simulink model "final_output"  (R2024a)
settings: Solver=VariableStepAuto  StartTime=0.0  StopTime=2  MaxStep=1e-3  RelTol=1e-3  EnableMultiTasking=on
PreLoadFcn:
  | DualActiveBridgeConverterData
values from neighbouring files (symbols this model uses):
  C_HV = 0.0001    [matlab.mat]
  C_LV = 0.002    [matlab.mat]
  Cs_FET = inf    [matlab.mat]
  Fsw = 100000    [matlab.mat]
  Ki_Ireg = 500    [matlab.mat]
  Kp_Ireg = 0.1    [matlab.mat]
  L_Inductor = 1.5e-05    [matlab.mat]
  Lm_Tr = 0.00072    [matlab.mat]
  Lprim_Tr = 1.7e-05    [matlab.mat]
  Lsec_Tr = 0    [matlab.mat]
  N_Tr = 1.6    [matlab.mat]
  Pnom = 10000    [matlab.mat]
  R_DCsrc1 = 0.01    [matlab.mat]
  R_DCsrc2 = 0.05    [matlab.mat]
  R_Inductor = 0.016    [matlab.mat]
  RC_HV = 0.001    [matlab.mat]
  RC_LV = 0.001    [matlab.mat]
  Rm_Tr = 10000    [matlab.mat]
  Ron_Diode = 0.01    [matlab.mat]
  Ron_FET = 0.016    [matlab.mat]
  Rprim_Tr = 0.043    [matlab.mat]
  Rs_FET = 1000000    [matlab.mat]
  Rsec_Tr = 1e-06    [matlab.mat]
  Ts_Control = 1e-06    [matlab.mat]
  Vf_Diode = 4.2    [matlab.mat]
  Vnom_HV = 800    [matlab.mat]
  Vnom_LV = 450    [matlab.mat]
undefined symbols (not defined in the file or in its folder): DiscIntNeverNeededParam, Ion, Lithium
libraries: spsSeriesRLCBranchLib x14, spsDiodeLib x12, spsVoltageMeasurementLib x11, spsMosfetLib x9, spsCurrentMeasurementLib x8, spsIdealSwitchLib x8, powerlib_extras x5, spsMeanLib x5, spsRMSLib x3, simulink x3, spsThreePhaseVIMeasurementLib x2, spsUniversalBridgeLib x2
(part 2 of 2)

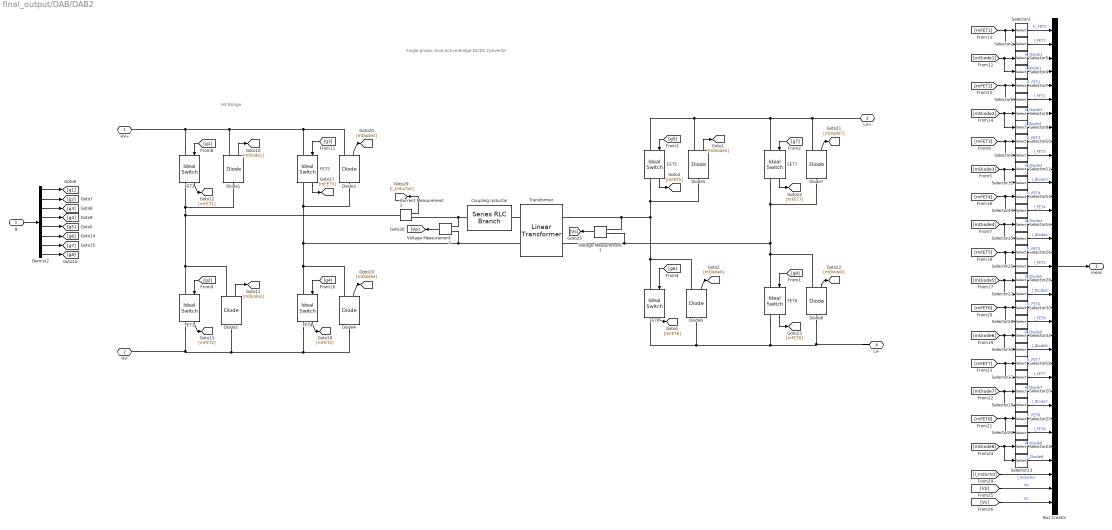
== system final_output/DAB/DAB2 ==
  note: HV Bridge
  note: Single-phase, Dual-Active Bridge
      | DC/DC Converter
  g : Inport  PortDimensions=8
  Bus Creator : BusCreator  Inputs=35
  Coupling Inductor : spsSeriesRLCBranchLib/Series RLC Branch  LConnTagsString=__new0  RConnTagsString=__new0  BranchType=RL  Resistance=R_Inductor  Inductance=L_Inductor  SetiL0=off  InitialCurrent=0  Capacitance=1e-6  Setx0=off  InitialVoltage=0  Measurements=None
  Current Measurement2 : spsCurrentMeasurementLib/Current Measurement  PhasorSimulation=off  OutputType=Complex  PSBequivalent=0
  Demux2 : Demux  Outputs=8
  Diode{1..8} (8 alike) : spsDiodeLib/Diode  Ron=Ron_Diode  Lon=0  Vf=Vf_Diode  IC=0  UseSnubber=0  Rs=inf  Cs=inf  Measurements=on
  FET{1..8} (8 alike) : spsIdealSwitchLib/Ideal Switch  Ron=Ron_FET  Lon=0  IC=0  Rs=Rs_FET  Cs=Cs_FET  Measurements=on
  Selector{1..2,4,6,8,11,13,15,17,19,21,23,25,27,29,31} (16 alike) : Selector  InputPortWidth=2  IndexOptions=Index vector (dialog)  Indices=1  OutputSizes=1
  Selector{3,5,7,9..10,12,14,16,18,20,22,24,26,28,30,32} (16 alike) : Selector  InputPortWidth=2  IndexOptions=Index vector (dialog)  Indices=2  OutputSizes=1
  Transformer : spsLinearTransformerLib/Linear Transformer  UNITS=SI  NominalPower="[ Param1_Tr(1),  Param1_Tr(2)]"  winding1="[ Param2_Tr(1),  Param2_Tr(2), Param2_Tr(3)]"  winding2="[ Param3_Tr(1),  Param3_Tr(2), Param3_Tr(3)]"  ThreeWindings=off  winding3=[3.15e+05 0.7938 0.084225]  RmLm="[ Param4_Tr(1),  Param4_Tr(2)]"  Measurements=None  DataType=on
  Voltage Measurement1 : spsVoltageMeasurementLib/Voltage Measurement  PhasorSimulation=off  OutputType=Complex  PSBequivalent=0
  Voltage Measurement2 : spsVoltageMeasurementLib/Voltage Measurement  PhasorSimulation=off  OutputType=Complex  PSBequivalent=0
  HV+ : PMIOPort  Side=Left
  HV- : PMIOPort  Port=2  Side=Left
  LV+ : PMIOPort  Port=3  Side=Right
  LV- : PMIOPort  Port=4  Side=Right
  meas : Outport  PortDimensions=35
  wires:
  Voltage Measurement2/1 -> [Vp]
  Demux2/8 -> [g8]
  Selector20/1 -> Bus Creator/27  "V_Diode7"
  Selector21/1 -> Bus Creator/30  "I_FET8"
  Selector22/1 -> Bus Creator/29  "V_FET8"
  Selector24/1 -> Bus Creator/31  "V_Diode8"
  [mDiode5] -> Selector27/1, Selector28/1
  Selector27/1 -> Bus Creator/20  "I_Diode5"
  [mFET6] -> Selector30/1, Selector29/1
  Selector23/1 -> Bus Creator/32  "I_Diode8"
  Selector32/1 -> Bus Creator/23  "V_Diode6"
  Selector26/1 -> Bus Creator/17  "V_FET5"
  Selector28/1 -> Bus Creator/19  "V_Diode5"
  Selector25/1 -> Bus Creator/18  "I_FET5"
  [mFET5] -> Selector25/1, Selector26/1
  FET3/1 -> [mFET3]
  Diode4/1 -> [mDiode4]
  FET4/1 -> [mFET4]
  Selector19/1 -> Bus Creator/28  "I_Diode7"
  FET7/1 -> [mFET7]
  Selector5/1 -> Bus Creator/3  "V_Diode1"
  [mDiode2] -> Selector8/1, Selector9/1
  [g4] -> FET4/1
  Selector4/1 -> Bus Creator/4  "I_Diode1"
  [mFET4] -> Selector14/1, Selector13/1
  Diode2/1 -> [mDiode2]
  Demux2/1 -> [g1]
  FET1/1 -> [mFET1]
  Selector18/1 -> Bus Creator/25  "V_FET7"
  Selector3/1 -> Bus Creator/1  "V_FET1"
  [mFET8] -> Selector21/1, Selector22/1
  FET2/1 -> [mFET2]
  [mDiode4] -> Selector16/1, Selector15/1
  [g1] -> FET1/1
  [g3] -> FET3/1
  Demux2/4 -> [g4]
  [mFET1] -> Selector3/1, Selector2/1
  Diode1/1 -> [mDiode1]
  Demux2/2 -> [g2]
  Diode6/1 -> [mDiode6]
  Demux2/3 -> [g3]
  Diode5/1 -> [mDiode5]
  [mDiode1] -> Selector5/1, Selector4/1
  Diode3/1 -> [mDiode3]
  Demux2/7 -> [g7]
  Selector6/1 -> Bus Creator/6  "I_FET2"
  Selector2/1 -> Bus Creator/2  "I_FET1"
  [mDiode3] -> Selector11/1, Selector12/1
  Selector13/1 -> Bus Creator/14  "I_FET4"
  Selector10/1 -> Bus Creator/9  "V_FET3"
  [mFET3] -> Selector1/1, Selector10/1
  Selector15/1 -> Bus Creator/16  "I_Diode4"
  Selector16/1 -> Bus Creator/15  "V_Diode4"
  Selector14/1 -> Bus Creator/13  "V_FET4"
  Selector30/1 -> Bus Creator/21  "V_FET6"
  [g7] -> FET7/1
  Demux2/6 -> [g6]
  [g8] -> FET8/1
  Selector9/1 -> Bus Creator/7  "V_Diode2"
  [g2] -> FET2/1
  FET6/1 -> [mFET6]
  Diode7/1 -> [mDiode7]
  [mDiode7] -> Selector20/1, Selector19/1
  Selector11/1 -> Bus Creator/12  "I_Diode3"
  Selector29/1 -> Bus Creator/22  "I_FET6"
  [mFET2] -> Selector6/1, Selector7/1
  [mDiode8] -> Selector23/1, Selector24/1
  Diode8/1 -> [mDiode8]
  FET5/1 -> [mFET5]
  Selector17/1 -> Bus Creator/26  "I_FET7"
  Selector12/1 -> Bus Creator/11  "V_Diode3"
  Current Measurement2/1 -> [I_Inductor]
  Selector1/1 -> Bus Creator/10  "I_FET3"
  Demux2/5 -> [g5]
  Selector31/1 -> Bus Creator/24  "I_Diode6"
  [mFET7] -> Selector18/1, Selector17/1
  Selector8/1 -> Bus Creator/8  "I_Diode2"
  [g5] -> FET5/1
  Selector7/1 -> Bus Creator/5  "V_FET2"
  FET8/1 -> [mFET8]
  [mDiode6] -> Selector32/1, Selector31/1
  [g6] -> FET6/1
  g/1 -> Demux2/1
  Bus Creator/1 -> meas/1
  Voltage Measurement1/1 -> [Vs]
  [I_Inductor] -> Bus Creator/33  "I_Inductor"
  [Vp] -> Bus Creator/34  "Vp"
  [Vs] -> Bus Creator/35  "Vs"
  connections:
  FET7/LConn1 -- LV+/RConn1 -- Diode7/RConn1 -- Diode5/RConn1 -- FET5/LConn1
  FET1/LConn1 -- HV+/RConn1 -- Diode3/RConn1 -- FET3/LConn1 -- Diode1/RConn1
  FET2/RConn1 -- HV-/RConn1 -- FET4/RConn1 -- Diode4/LConn1 -- Diode2/LConn1
  Diode2/RConn1 -- Current Measurement2/LConn1 -- Diode1/LConn1 -- FET1/RConn1 -- FET2/LConn1
  Diode4/RConn1 -- FET4/LConn1 -- Transformer/LConn2 -- Voltage Measurement2/LConn2 -- FET3/RConn1 -- Diode3/LConn1
  FET6/RConn1 -- Diode6/LConn1 -- LV-/RConn1 -- Diode8/LConn1 -- FET8/RConn1
  FET7/RConn1 -- Voltage Measurement1/LConn2 -- Transformer/RConn2 -- FET8/LConn1 -- Diode8/RConn1 -- Diode7/LConn1
  FET6/LConn1 -- Voltage Measurement1/LConn1 -- Transformer/RConn1 -- Diode5/LConn1 -- FET5/RConn1 -- Diode6/RConn1
  Current Measurement2/RConn1 -- Voltage Measurement2/LConn1 -- Coupling Inductor/LConn1
  Transformer/LConn1 -- Coupling Inductor/RConn1

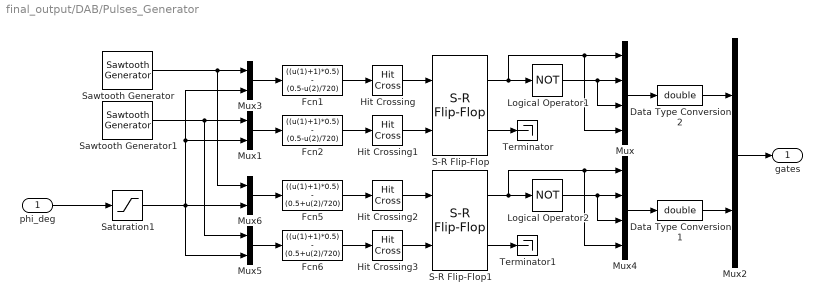
== system final_output/DAB/Pulses_Generator ==
  phi_deg : Inport
  Data Type Conversion1 : DataTypeConversion  OutDataTypeStr=double  SaturateOnIntegerOverflow=off  RndMeth=Floor
  Data Type Conversion2 : DataTypeConversion  OutDataTypeStr=double  SaturateOnIntegerOverflow=off  RndMeth=Floor
  Fcn1 : Fcn  Expr=((u(1)+1)*0.5) - (0.5-u(2)/720)
  Fcn2 : Fcn  Expr=((u(1)+1)*0.5) - (0.5-u(2)/720)
  Fcn5 : Fcn  Expr=((u(1)+1)*0.5) - (0.5+u(2)/720)
  Fcn6 : Fcn  Expr=((u(1)+1)*0.5) - (0.5+u(2)/720)
  Hit Crossing{,1..3} (4 alike) : HitCross  HitCrossingDirection=rising
  Logical Operator1 : Logic  Operator=NOT  AllPortsSameDT=off  OutDataTypeStr=boolean
  Logical Operator2 : Logic  Operator=NOT  AllPortsSameDT=off  OutDataTypeStr=boolean
  Mux : Mux
  Mux{1,3,5..6} (4 alike) : Mux  Inputs=2
  Mux2 : Mux  Inputs=[4,4]
  Mux4 : Mux
  S-R Flip-Flop : simulink_extras/Flip Flops/S-R Flip-Flop  initial_condition=0
  S-R Flip-Flop1 : simulink_extras/Flip Flops/S-R Flip-Flop  initial_condition=0
  Saturation1 : Saturate  UpperLimit=180  LowerLimit=-180
  Sawtooth Generator : spsSawtoothGeneratorLib/Sawtooth Generator  Freq=Fsw  Phase=0  Ts=0
  Sawtooth Generator1 : spsSawtoothGeneratorLib/Sawtooth Generator  Freq=Fsw  Phase=180  Ts=0
  Terminator : Terminator
  Terminator1 : Terminator
  gates : Outport
  wires:
  Mux2/1 -> gates/1
  Logical Operator1/1 -> Mux/2, Mux/3
  phi_deg/1 -> Saturation1/1
  Sawtooth Generator/1 -> Mux6/1, Mux3/1
  Fcn1/1 -> Hit Crossing/1
  Fcn2/1 -> Hit Crossing1/1
  Hit Crossing/1 -> S-R Flip-Flop/1
  Hit Crossing1/1 -> S-R Flip-Flop/2
  S-R Flip-Flop/1 -> Mux/4, Mux/1, Logical Operator1/1
  S-R Flip-Flop/2 -> Terminator/1
  Mux/1 -> Data Type Conversion2/1
  Data Type Conversion2/1 -> Mux2/1
  Data Type Conversion1/1 -> Mux2/2
  Mux3/1 -> Fcn1/1
  Mux1/1 -> Fcn2/1
  Sawtooth Generator1/1 -> Mux5/1, Mux1/1
  Saturation1/1 -> Mux6/2, Mux5/2, Mux1/2, Mux3/2
  Mux5/1 -> Fcn6/1
  Mux6/1 -> Fcn5/1
  Mux4/1 -> Data Type Conversion1/1
  S-R Flip-Flop1/2 -> Terminator1/1
  S-R Flip-Flop1/1 -> Logical Operator2/1, Mux4/1, Mux4/4
  Hit Crossing3/1 -> S-R Flip-Flop1/2
  Hit Crossing2/1 -> S-R Flip-Flop1/1
  Fcn6/1 -> Hit Crossing3/1
  Fcn5/1 -> Hit Crossing2/1
  Logical Operator2/1 -> Mux4/3, Mux4/2

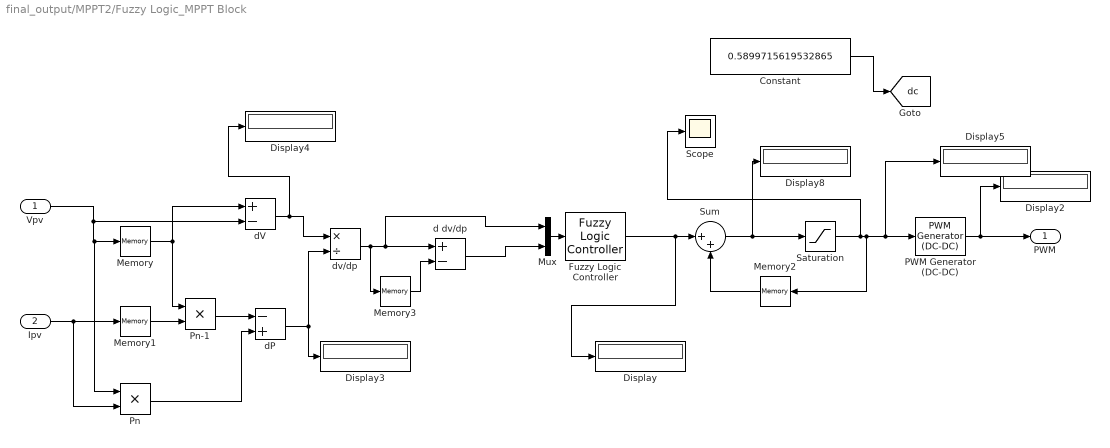
== system final_output/MPPT2/Fuzzy Logic_MPPT Block ==
  Vpv : Inport
  Ipv : Inport  Port=2
  Constant : Constant  Value=0.5899715619532865
  Display{,2..5,8} (6 alike) : Display
  Fuzzy Logic Controller : fuzblock/Fuzzy Logic  Controller  FIS='fuzzy_mppt.fis'  OutputSampleNumber=101  DataType=double  FuzzifiedInputs=off  RuleFiringStrengths=off  RuleOutputs=off  AggregatedOutputs=off  SimulateUsing=Interpreted execution  OutOfRangeInputValueMessage=warning  NoRuleFiredMessage=warning  EmptyOutputFuzzySetMessage=warning
  Memory{,1..3} (4 alike) : Memory  InheritSampleTime=on
  Mux : Mux  Inputs=2
  PWM Generator (DC-DC) : spsPWMGeneratorDCDCLib/PWM Generator (DC-DC)  Fsw=10000  Ts=0
  Pn : Product
  Pn-1 : Product
  Saturation : Saturate  UpperLimit=0.9  LowerLimit=0.1  OutDataTypeStr=double
  Scope : Scope
  Sum : Sum  Inputs=|++
  d dv/dp : Sum  Inputs=+-
  dP : Sum  Inputs=-+
  dV : Sum  Inputs=+-
  dv/dp : Product  Inputs=*/
  PWM : Outport  VectorParamsAs1DForOutWhenUnconnected=off
  tag scope: dc=global
  wires:
  Vpv/1 -> Memory/1, Pn/1, dV/2
  PWM Generator (DC-DC)/1 -> PWM/1, Display2/1
  Mux/1 -> Fuzzy Logic Controller/1
  Pn/1 -> dP/2
  Pn-1/1 -> dP/1
  Memory1/1 -> Pn-1/2
  Ipv/1 -> Memory1/1, Pn/2
  Memory/1 -> Pn-1/1, dV/1
  dV/1 -> Display4/1, dv/dp/1
  dP/1 -> dv/dp/2, Display3/1
  dv/dp/1 -> Memory3/1, Mux/1, d dv/dp/1
  Memory3/1 -> d dv/dp/2
  Memory2/1 -> Sum/2
  Sum/1 -> Display8/1, Saturation/1
  Constant/1 -> [dc]
  d dv/dp/1 -> Mux/2
  Saturation/1 -> Display5/1, PWM Generator (DC-DC)/1, Memory2/1, Scope/1
  Fuzzy Logic Controller/1 -> Sum/1, Display/1

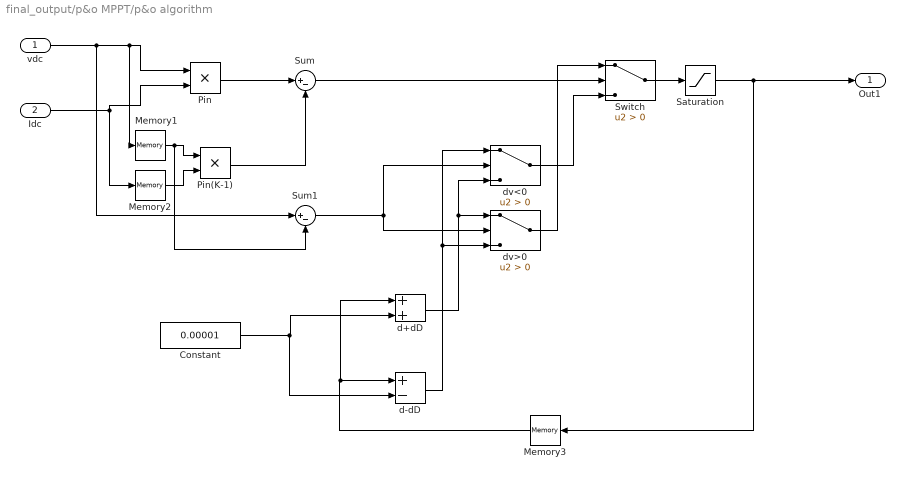
== system final_output/p&o MPPT/p&o algorithm ==
  vdc : Inport
  Idc : Inport  Port=2
  Constant : Constant  Value=0.00001
  Memory1 : Memory
  Memory2 : Memory
  Memory3 : Memory
  Pin : Product
  Pin(K-1) : Product
  Saturation : Saturate  UpperLimit=0.9  LowerLimit=0
  Sum : Sum  Inputs=|+-
  Sum1 : Sum  Inputs=|+-
  Switch : Switch  Criteria=u2 > Threshold  SaturateOnIntegerOverflow=off  InputSameDT=off
  d+dD : Sum
  d-dD : Sum  Inputs=+-
  dv<0 : Switch  Criteria=u2 > Threshold  SaturateOnIntegerOverflow=off  InputSameDT=off
  dv>0 : Switch  Criteria=u2 > Threshold  SaturateOnIntegerOverflow=off  InputSameDT=off
  Out1 : Outport
  wires:
  vdc/1 -> Sum1/1, Memory1/1, Pin/1
  Idc/1 -> Pin/2, Memory2/1
  Memory1/1 -> Sum1/2, Pin(K-1)/1
  Memory2/1 -> Pin(K-1)/2
  Pin/1 -> Sum/1
  Pin(K-1)/1 -> Sum/2
  Sum/1 -> Switch/2
  Sum1/1 -> dv<0/2, dv>0/2
  dv<0/1 -> Switch/3
  Memory3/1 -> d+dD/1, d-dD/1
  Switch/1 -> Saturation/1
  Constant/1 -> d-dD/2, d+dD/2
  d+dD/1 -> dv<0/3, dv>0/1
  d-dD/1 -> dv>0/3, dv<0/1
  dv>0/1 -> Switch/1
  Saturation/1 -> Memory3/1, Out1/1

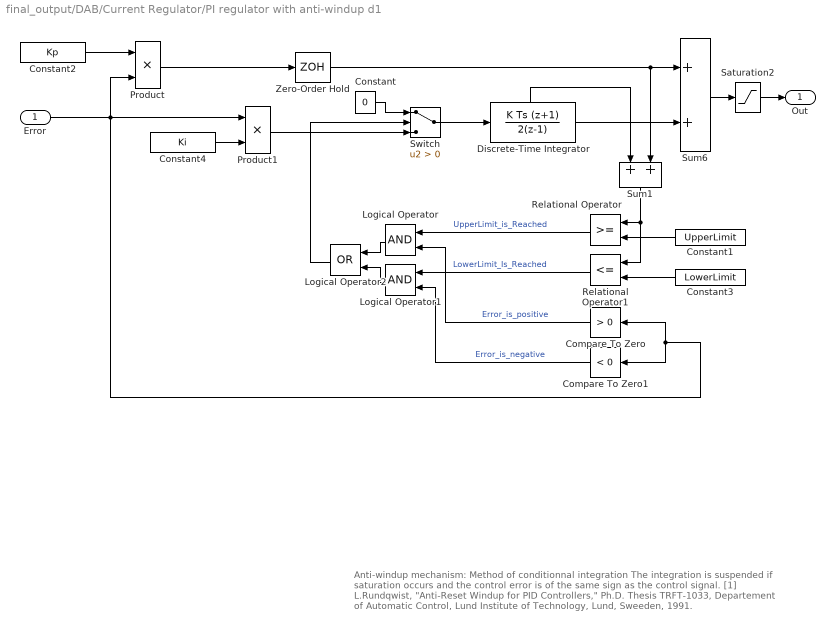
== system final_output/DAB/Current Regulator/PI regulator with anti-windup d1 ==
  note: Anti-windup mechanism: Method of conditionnal integration
      |
      | The integration is suspended if saturation occurs and the
      | control error is of the same sign as the control signal.
      |
      | [1] L.Rundqwist, "Anti-Reset Windup for PID Controllers," Ph.D. Thesis TRFT-1033,
      | Departement of Automatic Control, Lund Institute of Technology, Lund, Sweeden, 1991.
  Error : Inport  SampleTime=Ts
  Compare To Zero : simulink/Logic and Bit Operations/Compare To Zero  relop=>  OutDataTypeStr=uint8  ZeroCross=off
  Compare To Zero1 : simulink/Logic and Bit Operations/Compare To Zero  relop=<  OutDataTypeStr=uint8  ZeroCross=off
  Constant : Constant  Value=0
  Constant1 : Constant  Value=UpperLimit
  Constant2 : Constant  Value=Kp  SampleTime=Ts
  Constant3 : Constant  Value=LowerLimit
  Constant4 : Constant  Value=Ki  SampleTime=Ts
  Discrete-Time Integrator : DiscreteIntegrator  IntegratorMethod=Integration: Trapezoidal  InitialCondition=Init  SampleTime=Ts  LimitOutput=on  UpperSaturationLimit=UpperLimit  LowerSaturationLimit=LowerLimit  ShowStatePort=on  ICPrevOutput=DiscIntNeverNeededParam  ICPrevScaledInput=DiscIntNeverNeededParam
  Logical Operator : Logic  AllPortsSameDT=off  OutDataTypeStr=boolean
  Logical Operator1 : Logic  AllPortsSameDT=off  OutDataTypeStr=boolean
  Logical Operator2 : Logic  Operator=OR  AllPortsSameDT=off  OutDataTypeStr=boolean
  Product : Product
  Product1 : Product
  Relational Operator : RelationalOperator  OutDataTypeStr=boolean  InputSameDT=off
  Relational Operator1 : RelationalOperator  Operator=<=  OutDataTypeStr=boolean  InputSameDT=off
  Saturation2 : Saturate  UpperLimit=UpperLimit  LowerLimit=LowerLimit  SampleTime=Ts
  Sum1 : Sum  InputSameDT=on  SaturateOnIntegerOverflow=on  SampleTime=Ts  OutDataTypeStr=Inherit: Same as first input
  Sum6 : Sum  InputSameDT=on  SaturateOnIntegerOverflow=on  SampleTime=Ts  OutDataTypeStr=Inherit: Same as first input
  Switch : Switch  Criteria=u2 > Threshold  SaturateOnIntegerOverflow=off  InputSameDT=off
  Zero-Order Hold : ZeroOrderHold  SampleTime=Ts
  Out : Outport  SampleTime=Ts  InitialOutput=0  VectorParamsAs1DForOutWhenUnconnected=off
  wires:
  Constant2/1 -> Product/1
  Product1/1 -> Switch/3
  Switch/1 -> Discrete-Time Integrator/1
  Saturation2/1 -> Out/1
  Discrete-Time Integrator/1 -> Sum6/2
  Product/1 -> Zero-Order Hold/1
  Sum6/1 -> Saturation2/1
  Error/1 -> Product1/1, Product/2, Compare To Zero/1, Compare To Zero1/1
  Compare To Zero1/1 -> Logical Operator1/2  "Error_is_negative"
  Logical Operator1/1 -> Logical Operator2/2
  Logical Operator/1 -> Logical Operator2/1
  Compare To Zero/1 -> Logical Operator/2  "Error_is_positive"
  Constant3/1 -> Relational Operator1/2
  Constant1/1 -> Relational Operator/2
  Relational Operator1/1 -> Logical Operator1/1  "LowerLimit_Is_Reached"
  Relational Operator/1 -> Logical Operator/1  "UpperLimit_is_Reached"
  Logical Operator2/1 -> Switch/2
  Sum1/1 -> Relational Operator/1, Relational Operator1/1
  Discrete-Time Integrator/State -> Sum1/1
  Zero-Order Hold/1 -> Sum6/1, Sum1/2
  Constant/1 -> Switch/1
  Constant4/1 -> Product1/2
